simulink model "E1_VehiculoAereo1DOFsim"  (R2016b)
settings: Solver=ode4  StartTime=0.0  StopTime=120  FixedStep=dt  RelTol=1e-3  EnableMultiTasking=on
values from neighbouring files (symbols this model uses):
  B = 0.162    [Ejercicio1.m]
  COlim = [0 10]    [Ejercicio1.m]
  COnom = Fpnom/Kt    (= 5)    [Ejercicio1.m]
  dt = 0.002    [Ejercicio1.m]
  Fpdotlim = [-1 1]*16e3/5    [Ejercicio1.m]
  Fplim = [0 1]*16e3    [Ejercicio1.m]
  Fpnom = 8e3    (= 8000)    [Ejercicio1.m]
  Kd = 5    [Ejercicio1.m]
  Ki = 0.5    [Ejercicio1.m]
  Km = 10/300    (= 0.0333333333333)    [Ejercicio1.m]
  Kp = 5    [Ejercicio1.m]
  Kt = 16e3/10    (= 1600)    [Ejercicio1.m]
  m = 400    [Ejercicio1.m]
  tauf = 0.02    [Ejercicio1.m]
  taufd = Kd/10    (= 0.5)    [Ejercicio1.m]
  taum = 0.1    [Ejercicio1.m]
  taup = 1    [Ejercicio1.m]
  Vmfnom = Vmnom    (= 7.40740740741)    [Ejercicio1.m]
  Vmlim = [0 10]    [Ejercicio1.m]
  Vmnom = Vnom*Km    (= 7.40740740741)    [Ejercicio1.m]
  Vnom = 800*10/36    (= 222.222222222)    [Ejercicio1.m]
settings Model: Creator=Jairo  LastModifiedBy=elena
settings DataIOCC: LimitDataPoints=on  SaveFormat=Array
settings OptimizationCC: LifeSpan=inf
settings DebuggingCC: SolverPrmCheckMsg=warning  SFUnexpectedBacktrackingDiag=warning  SFNoUnconditionalDefaultTransitionDiag=warning  SFExecutionAtInitializationDiag=none
settings HardwareCC: ProdBitPerPointer=32  ProdBitPerSizeT=32  ProdBitPerPtrDiffT=32  ProdLargestAtomicFloat=None  ProdIntDivRoundTo=Undefined  ProdEndianess=Unspecified  ProdWordSize=32  ProdHWDeviceType=32-bit Generic
settings ModelReferenceCC: PropagateSignalLabelsOutOfModel=off
settings GRTTargetCC: TargetLangStandard=C89/C90 (ANSI)  GeneratePreprocessorConditionals=Disable all
settings ConfigComp: CovMetricSettings=dw  CovHtmlReporting=on  CovSaveCumulativeToWorkspaceVar=on  CovSaveSingleToWorkspaceVar=on  CovExternalEMLEnable=off  CovSFcnEnable=off

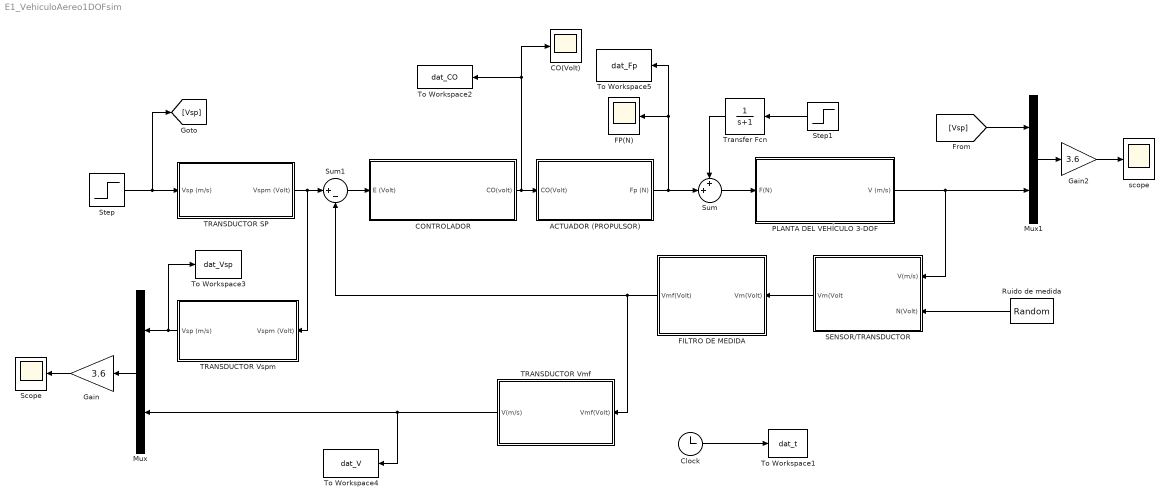
== system E1_VehiculoAereo1DOFsim ==
  ACTUADOR (PROPULSOR) : Subsystem
  CO(Volt) : Scope
  CONTROLADOR : Subsystem
  Clock : Clock
  FILTRO DE MEDIDA : Subsystem
  FP(N) : Scope
  Gain : Gain  Gain=3.6
  Gain2 : Gain  Gain=3.6
  Mux : Mux  Inputs=2
  Mux1 : Mux  Inputs=2
  PLANTA DEL VEHÍCULO 3-DOF : Subsystem
  Ruido de medida : RandomNumber  Variance=1e-5  Seed=123456  SampleTime=dt
  SENSOR/TRANSDUCTOR : Subsystem
  Scope : Scope
  Step : Step  Time=10  Before=Vnom  After=Vnom+50/3.6  SampleTime=0
  Step1 : Step  Time=60  After=-1e3  SampleTime=0
  Sum : Sum  Inputs=++|  SaturateOnIntegerOverflow=on
  Sum1 : Sum  Inputs=|+-
  TRANSDUCTOR SP : Subsystem
  TRANSDUCTOR Vmf : Subsystem
  TRANSDUCTOR Vspm : Subsystem
  To Workspace1 : ToWorkspace  VariableName=dat_t  SampleTime=-1
  To Workspace2 : ToWorkspace  VariableName=dat_CO  SampleTime=-1
  To Workspace3 : ToWorkspace  VariableName=dat_Vsp  SampleTime=-1
  To Workspace4 : ToWorkspace  VariableName=dat_V  SampleTime=-1
  To Workspace5 : ToWorkspace  VariableName=dat_Fp  SampleTime=-1
  Transfer Fcn : TransferFcn  Denominator=[1 1]
  scope : Scope
  wires:
  CONTROLADOR/1(CO(volt)) -> CO(Volt)/1, To Workspace2/1, ACTUADOR (PROPULSOR)/1(CO(Volt))
  ACTUADOR (PROPULSOR)/1(Fp (N)) -> To Workspace5/1, FP(N)/1, Sum/2
  SENSOR/TRANSDUCTOR/1(Vm(Volt) -> FILTRO DE MEDIDA/1(Vm(Volt))
  Sum1/1 -> CONTROLADOR/1(E (Volt))
  FILTRO DE MEDIDA/1(Vmf(Volt)) -> TRANSDUCTOR Vmf/1(Vmf(Volt)), Sum1/2
  TRANSDUCTOR SP/1(Vspm (Volt)) -> TRANSDUCTOR Vspm/1(Vspm (Volt)), Sum1/1
  TRANSDUCTOR Vspm/1(Vsp (m/s)) -> To Workspace3/1, Mux/1
  TRANSDUCTOR Vmf/1(V(m/s)) -> To Workspace4/1, Mux/2
  Mux/1 -> Gain/1
  Gain/1 -> Scope/1
  Ruido de medida/1 -> SENSOR/TRANSDUCTOR/2(N(Volt))
  Step/1 -> [Vsp], TRANSDUCTOR SP/1(Vsp (m/s))
  [Vsp] -> Mux1/1
  PLANTA DEL VEHÍCULO 3-DOF/1(V (m/s)) -> SENSOR/TRANSDUCTOR/1(V(m/s)), Mux1/2
  Clock/1 -> To Workspace1/1
  Transfer Fcn/1 -> Sum/1
  Step1/1 -> Transfer Fcn/1
  Sum/1 -> PLANTA DEL VEHÍCULO 3-DOF/1(F(N))
  Mux1/1 -> Gain2/1
  Gain2/1 -> scope/1

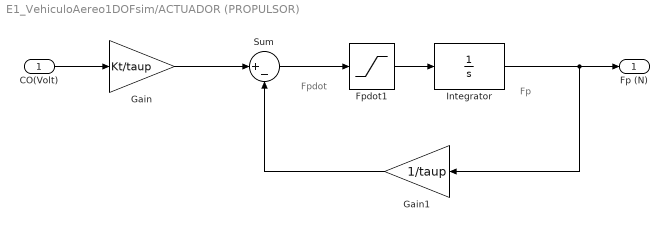
== system E1_VehiculoAereo1DOFsim/ACTUADOR (PROPULSOR) ==
  note: Fp
  note: Fpdot
  CO(Volt) : Inport
  Fpdot1 : Saturate  UpperLimit=Fpdotlim(2)  LowerLimit=Fpdotlim(1)
  Gain : Gain  Gain=Kt/taup
  Gain1 : Gain  Gain=1/taup
  Integrator : Integrator  InitialCondition=Fpnom  LimitOutput=on  UpperSaturationLimit=Fplim(2)  LowerSaturationLimit=Fplim(1)
  Sum : Sum  Inputs=|+-
  Fp (N) : Outport
  wires:
  CO(Volt)/1 -> Gain/1
  Gain/1 -> Sum/1
  Sum/1 -> Fpdot1/1
  Fpdot1/1 -> Integrator/1
  Integrator/1 -> Fp (N)/1, Gain1/1
  Gain1/1 -> Sum/2

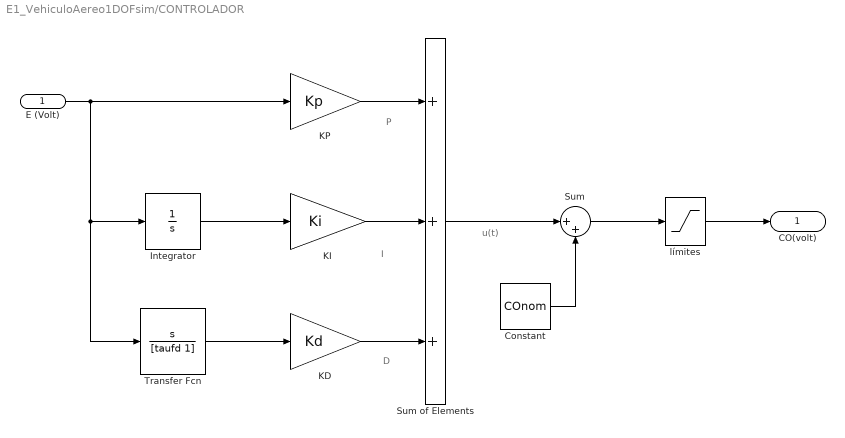
== system E1_VehiculoAereo1DOFsim/CONTROLADOR ==
  note: u(t)
  note: D
  note: I
  note: P
  E (Volt) : Inport
  Constant : Constant  Value=COnom
  Integrator : Integrator
  KD : Gain  Gain=Kd
  KI : Gain  Gain=Ki
  KP : Gain  Gain=Kp
  Sum : Sum  Inputs=|++
  Sum of Elements : Sum  Inputs=+++
  Transfer Fcn : TransferFcn  Numerator=[1 0]  Denominator=[taufd 1]
  límites : Saturate  UpperLimit=COlim(2)  LowerLimit=COlim(1)
  CO(volt) : Outport
  wires:
  Integrator/1 -> KI/1
  E (Volt)/1 -> Transfer Fcn/1, Integrator/1, KP/1
  Transfer Fcn/1 -> KD/1
  Sum of Elements/1 -> Sum/1
  Constant/1 -> Sum/2
  Sum/1 -> límites/1
  límites/1 -> CO(volt)/1
  KP/1 -> Sum of Elements/1
  KD/1 -> Sum of Elements/3
  KI/1 -> Sum of Elements/2

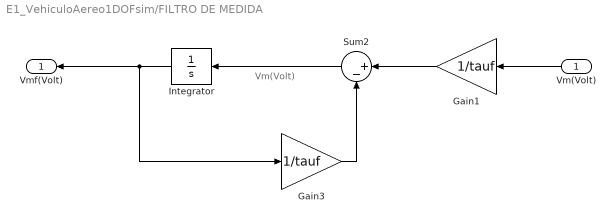
== system E1_VehiculoAereo1DOFsim/FILTRO DE MEDIDA ==
  note: Vm(Volt)
  Vm(Volt) : Inport
  Gain1 : Gain  Gain=1/tauf
  Gain3 : Gain  Gain=1/tauf
  Integrator : Integrator  InitialCondition=Vmfnom
  Sum2 : Sum  Inputs=|+-
  Vmf(Volt) : Outport
  wires:
  Vm(Volt)/1 -> Gain1/1
  Gain1/1 -> Sum2/1
  Sum2/1 -> Integrator/1
  Gain3/1 -> Sum2/2
  Integrator/1 -> Vmf(Volt)/1, Gain3/1

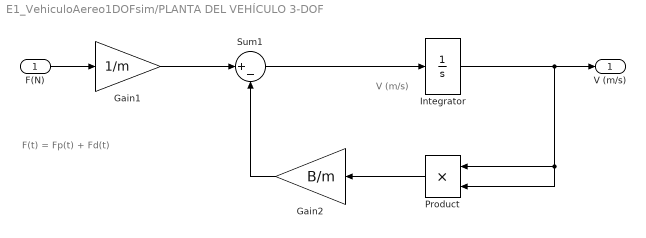
== system E1_VehiculoAereo1DOFsim/PLANTA DEL VEHÍCULO 3-DOF ==
  note: F(t) = Fp(t) + Fd(t)
  note: V (m/s)
  F(N) : Inport
  Gain1 : Gain  Gain=1/m
  Gain2 : Gain  Gain=B/m
  Integrator : Integrator  InitialCondition=Vnom
  Product : Product
  Sum1 : Sum  Inputs=|+-
  V (m/s) : Outport
  wires:
  F(N)/1 -> Gain1/1
  Gain1/1 -> Sum1/1
  Sum1/1 -> Integrator/1
  Gain2/1 -> Sum1/2
  Integrator/1 -> V (m/s)/1, Product/2, Product/1
  Product/1 -> Gain2/1

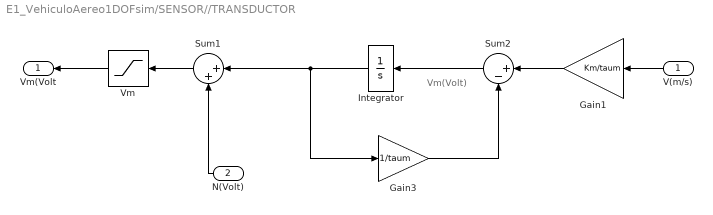
== system E1_VehiculoAereo1DOFsim/SENSOR//TRANSDUCTOR ==
  note: Vm(Volt)
  V(m/s) : Inport
  N(Volt) : Inport  Port=2
  Gain1 : Gain  Gain=Km/taum
  Gain3 : Gain  Gain=1/taum
  Integrator : Integrator  InitialCondition=Vmnom
  Sum1 : Sum  Inputs=|++
  Sum2 : Sum  Inputs=|+-
  Vm : Saturate  UpperLimit=Vmlim(2)  LowerLimit=Vmlim(1)
  Vm(Volt : Outport
  wires:
  V(m/s)/1 -> Gain1/1
  Gain1/1 -> Sum2/1
  Sum2/1 -> Integrator/1
  Integrator/1 -> Gain3/1, Sum1/1
  N(Volt)/1 -> Sum1/2
  Gain3/1 -> Sum2/2
  Sum1/1 -> Vm/1
  Vm/1 -> Vm(Volt/1

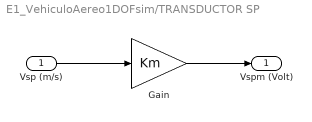
== system E1_VehiculoAereo1DOFsim/TRANSDUCTOR SP ==
  Vsp (m/s) : Inport
  Gain : Gain  Gain=Km
  Vspm (Volt) : Outport
  wires:
  Vsp (m/s)/1 -> Gain/1
  Gain/1 -> Vspm (Volt)/1

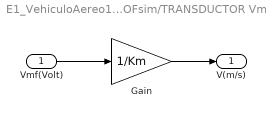
== system E1_VehiculoAereo1DOFsim/TRANSDUCTOR Vmf ==
  Vmf(Volt) : Inport
  Gain : Gain  Gain=1/Km  SaturateOnIntegerOverflow=on  OutDataTypeStr=Inherit: Same as input  ParamDataTypeStr=Inherit: Same as input
  V(m/s) : Outport
  wires:
  Vmf(Volt)/1 -> Gain/1
  Gain/1 -> V(m/s)/1

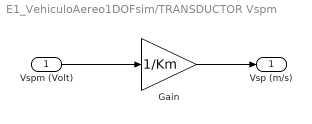
== system E1_VehiculoAereo1DOFsim/TRANSDUCTOR Vspm ==
  Vspm (Volt) : Inport
  Gain : Gain  Gain=1/Km
  Vsp (m/s) : Outport
  wires:
  Vspm (Volt)/1 -> Gain/1
  Gain/1 -> Vsp (m/s)/1
